simulink library "inp"  (R2021b)
settings: Solver=VariableStepAuto  StartTime=0.0  StopTime=10.0  RelTol=1e-3
undefined symbols (not defined in the file): C_TASK_5MS_S, FALSE, KINP_AcoreReadyToSlp_flg_ovrdflg, KINP_AcoreReadyToSlp_flg_ovrdval, KINP_AllowMovThd_OTA_enum_ovrdflg, KINP_AllowMovThd_OTA_enum_ovrdval, KINP_APSAngleTarget_Deg_ovrdflg, KINP_APSAngleTarget_Deg_ovrdval, KINP_APSDecReq_mps2_ovrdflg, KINP_APSDecReq_mps2_ovrdval, KINP_APSDecReqA_flg_ovrdflg, KINP_APSDecReqA_flg_ovrdval, KINP_APSDFLL_cm_ovrdflg, KINP_APSDFLL_cm_ovrdval, KINP_APSDFLR_cm_ovrdflg, KINP_APSDFLR_cm_ovrdval, KINP_APSDRLL_cm_ovrdflg, KINP_APSDRLL_cm_ovrdval, KINP_APSDRLR_cm_ovrdflg, KINP_APSDRLR_cm_ovrdval, KINP_APSExitCondition_enum_ovrdflg, KINP_APSExitCondition_enum_ovrdval, KINP_APSHWVer_enum_ovrdflg, KINP_APSHWVer_enum_ovrdval, KINP_APSProgressPCT_pct_ovrdflg, KINP_APSProgressPCT_pct_ovrdval, KINP_APSReq_enum_ovrdflg, KINP_APSReq_enum_ovrdval, KINP_APSRQDisplay_enum_ovrdflg, KINP_APSRQDisplay_enum_ovrdval, KINP_APSRqEPASCtrl_flg_ovrdflg, KINP_APSRqEPASCtrl_flg_ovrdval, KINP_APSShiftPosnReq_enum_ovrdval, KINP_APSShiftPosnReq_enum_ovrflg, KINP_APSSpeedCMD_kph_ovrdval, KINP_APSSpeedCMD_kph_ovrflg, KINP_APSStaSystem_enum_ovrdflg, KINP_APSStaSystem_enum_ovrdval, KINP_APSSWVer_enum_ovrdflg, KINP_APSSWVer_enum_ovrdval, KINP_APSVMCReqA_flg_ovrdval, KINP_APSVMCReqA_flg_ovrflg, KINP_APSVRqEPASCtrl_flg_ovrdflg, KINP_APSVRqEPASCtrl_flg_ovrdval, KINP_AuxBattVolmV_mV_ovrdflg, KINP_AuxBattVolmV_mV_ovrdval, KINP_CAASSta_enum_ovrdflg, KINP_CAASSta_enum_ovrdval, KINP_CAASVMCReqA_flg_ovrdval, KINP_CAASVMCReqA_flg_ovrflg, KINP_Chime_enum_ovrdflg, KINP_Chime_enum_ovrdval, KINP_ClearDTCcmd_flg_ovrdflg, KINP_ClearDTCcmd_flg_ovrdval, KINP_EvccAplusPwrUpReq_flg_ovrdflg, KINP_EvccAplusPwrUpReq_flg_ovrdval, KINP_LFID_raw_ovrdval, KINP_LFID_raw_ovrflg, KINP_LRID_raw_ovrdval, KINP_MemOffsetAccX_raw16_ovrdflg ... (+118)
libraries: FVT_lib x595, hcu_lib x1
(part 10 of 27)

== system inp/INP/CAN1/SignalCheck/ESC3 ==
  BHAL_outputs : Inport
  inp_CanValid_bus : Inport  Port=2
  LRPulseCount : FVT_lib/inp/can_signal_template  SystemSampleTime=-1  VariantActivationTime=update diagram  Latency=0  AutoFrameSizeCalculation=off
      link override defval: Value=KINP_LRPulseCount_enum_defval
      link override fftdec: Value=KINP_LRPulseCount_enum_fftdec
      link override fftinc: Value=KINP_LRPulseCount_enum_fftinc
      link override fftlim: Value=KINP_LRPulseCount_enum_fftlim
      link override invalid: Value=KINP_LRPulseCount_enum_invalid
      link override ovrdflg: Value=KINP_LRPulseCount_enum_ovrdflg
      link override ovrdval: Value=KINP_LRPulseCount_enum_ovrdval
      link override setvalid: Value=KINP_LRPulseCount_enum_setvalid
      link override srvcflg: Value=KINP_LRPulseCount_enum_srvcflg
      link override srvcval: Value=KINP_LRPulseCount_enum_srvcval
  LRPulseCountV : FVT_lib/inp/can_signal_template  SystemSampleTime=-1  VariantActivationTime=update diagram  Latency=0  AutoFrameSizeCalculation=off
      link override defval: Value=KINP_LRPulseCountV_flg_defval
      link override fftdec: Value=KINP_LRPulseCountV_flg_fftdec
      link override fftinc: Value=KINP_LRPulseCountV_flg_fftinc
      link override fftlim: Value=KINP_LRPulseCountV_flg_fftlim
      link override invalid: Value=KINP_LRPulseCountV_flg_invalid
      link override ovrdflg: Value=KINP_LRPulseCountV_flg_ovrdflg
      link override ovrdval: Value=KINP_LRPulseCountV_flg_ovrdval
      link override setvalid: Value=KINP_LRPulseCountV_flg_setvalid
      link override srvcflg: Value=KINP_LRPulseCountV_flg_srvcflg
      link override srvcval: Value=KINP_LRPulseCountV_flg_srvcval
  LRRawWhlSpeed : FVT_lib/inp/can_signal_template  SystemSampleTime=-1  VariantActivationTime=update diagram  Latency=0  AutoFrameSizeCalculation=off
      link override defval: Value=KINP_LRRawWhlSpeed_kph_defval
      link override fftdec: Value=KINP_LRRawWhlSpeed_kph_fftdec
      link override fftinc: Value=KINP_LRRawWhlSpeed_kph_fftinc
      link override fftlim: Value=KINP_LRRawWhlSpeed_kph_fftlim
      link override invalid: Value=KINP_LRRawWhlSpeed_kph_invalid
      link override ovrdflg: Value=KINP_LRRawWhlSpeed_kph_ovrdflg
      link override ovrdval: Value=KINP_LRRawWhlSpeed_kph_ovrdval
      link override setvalid: Value=KINP_LRRawWhlSpeed_kph_setvalid
      link override srvcflg: Value=KINP_LRRawWhlSpeed_kph_srvcflg
      link override srvcval: Value=KINP_LRRawWhlSpeed_kph_srvcval
  LRRawWhlSpeedV : FVT_lib/inp/can_signal_template  SystemSampleTime=-1  VariantActivationTime=update diagram  Latency=0  AutoFrameSizeCalculation=off
      link override defval: Value=KINP_LRRawWhlSpeedV_flg_defval
      link override fftdec: Value=KINP_LRRawWhlSpeedV_flg_fftdec
      link override fftinc: Value=KINP_LRRawWhlSpeedV_flg_fftinc
      link override fftlim: Value=KINP_LRRawWhlSpeedV_flg_fftlim
      link override invalid: Value=KINP_LRRawWhlSpeedV_flg_invalid
      link override ovrdflg: Value=KINP_LRRawWhlSpeedV_flg_ovrdflg
      link override ovrdval: Value=KINP_LRRawWhlSpeedV_flg_ovrdval
      link override setvalid: Value=KINP_LRRawWhlSpeedV_flg_setvalid
      link override srvcflg: Value=KINP_LRRawWhlSpeedV_flg_srvcflg
      link override srvcval: Value=KINP_LRRawWhlSpeedV_flg_srvcval
  LRWhlRotDir : FVT_lib/inp/can_signal_template  SystemSampleTime=-1  VariantActivationTime=update diagram  Latency=0  AutoFrameSizeCalculation=off
      link override defval: Value=KINP_LRWhlRotDir_enum_defval
      link override fftdec: Value=KINP_LRWhlRotDir_enum_fftdec
      link override fftinc: Value=KINP_LRWhlRotDir_enum_fftinc
      link override fftlim: Value=KINP_LRWhlRotDir_enum_fftlim
      link override invalid: Value=KINP_LRWhlRotDir_enum_invalid
      link override ovrdflg: Value=KINP_LRWhlRotDir_enum_ovrdflg
      link override ovrdval: Value=KINP_LRWhlRotDir_enum_ovrdval
      link override setvalid: Value=KINP_LRWhlRotDir_enum_setvalid
      link override srvcflg: Value=KINP_LRWhlRotDir_enum_srvcflg
      link override srvcval: Value=KINP_LRWhlRotDir_enum_srvcval
  RRPulseCount : FVT_lib/inp/can_signal_template  SystemSampleTime=-1  VariantActivationTime=update diagram  Latency=0  AutoFrameSizeCalculation=off
      link override defval: Value=KINP_RRPulseCount_enum_defval
      link override fftdec: Value=KINP_RRPulseCount_enum_fftdec
      link override fftinc: Value=KINP_RRPulseCount_enum_fftinc
      link override fftlim: Value=KINP_RRPulseCount_enum_fftlim
      link override invalid: Value=KINP_RRPulseCount_enum_invalid
      link override ovrdflg: Value=KINP_RRPulseCount_enum_ovrdflg
      link override ovrdval: Value=KINP_RRPulseCount_enum_ovrdval
      link override setvalid: Value=KINP_RRPulseCount_enum_setvalid
      link override srvcflg: Value=KINP_RRPulseCount_enum_srvcflg
      link override srvcval: Value=KINP_RRPulseCount_enum_srvcval
  RRPulseCountV : FVT_lib/inp/can_signal_template  SystemSampleTime=-1  VariantActivationTime=update diagram  Latency=0  AutoFrameSizeCalculation=off
      link override defval: Value=KINP_RRPulseCountV_flg_defval
      link override fftdec: Value=KINP_RRPulseCountV_flg_fftdec
      link override fftinc: Value=KINP_RRPulseCountV_flg_fftinc
      link override fftlim: Value=KINP_RRPulseCountV_flg_fftlim
      link override invalid: Value=KINP_RRPulseCountV_flg_invalid
      link override ovrdflg: Value=KINP_RRPulseCountV_flg_ovrdflg
      link override ovrdval: Value=KINP_RRPulseCountV_flg_ovrdval
      link override setvalid: Value=KINP_RRPulseCountV_flg_setvalid
      link override srvcflg: Value=KINP_RRPulseCountV_flg_srvcflg
      link override srvcval: Value=KINP_RRPulseCountV_flg_srvcval
  RRRawWhlSpeed : FVT_lib/inp/can_signal_template  SystemSampleTime=-1  VariantActivationTime=update diagram  Latency=0  AutoFrameSizeCalculation=off
      link override defval: Value=KINP_RRRawWhlSpeed_kph_defval
      link override fftdec: Value=KINP_RRRawWhlSpeed_kph_fftdec
      link override fftinc: Value=KINP_RRRawWhlSpeed_kph_fftinc
      link override fftlim: Value=KINP_RRRawWhlSpeed_kph_fftlim
      link override invalid: Value=KINP_RRRawWhlSpeed_kph_invalid
      link override ovrdflg: Value=KINP_RRRawWhlSpeed_kph_ovrdflg
      link override ovrdval: Value=KINP_RRRawWhlSpeed_kph_ovrdval
      link override setvalid: Value=KINP_RRRawWhlSpeed_kph_setvalid
      link override srvcflg: Value=KINP_RRRawWhlSpeed_kph_srvcflg
      link override srvcval: Value=KINP_RRRawWhlSpeed_kph_srvcval
  RRRawWhlSpeedV : FVT_lib/inp/can_signal_template  SystemSampleTime=-1  VariantActivationTime=update diagram  Latency=0  AutoFrameSizeCalculation=off
      link override defval: Value=KINP_RRRawWhlSpeedV_flg_defval
      link override fftdec: Value=KINP_RRRawWhlSpeedV_flg_fftdec
      link override fftinc: Value=KINP_RRRawWhlSpeedV_flg_fftinc
      link override fftlim: Value=KINP_RRRawWhlSpeedV_flg_fftlim
      link override invalid: Value=KINP_RRRawWhlSpeedV_flg_invalid
      link override ovrdflg: Value=KINP_RRRawWhlSpeedV_flg_ovrdflg
      link override ovrdval: Value=KINP_RRRawWhlSpeedV_flg_ovrdval
      link override setvalid: Value=KINP_RRRawWhlSpeedV_flg_setvalid
      link override srvcflg: Value=KINP_RRRawWhlSpeedV_flg_srvcflg
      link override srvcval: Value=KINP_RRRawWhlSpeedV_flg_srvcval
  RRWhlRotDir : FVT_lib/inp/can_signal_template  SystemSampleTime=-1  VariantActivationTime=update diagram  Latency=0  AutoFrameSizeCalculation=off
      link override defval: Value=KINP_RRWhlRotDir_enum_defval
      link override fftdec: Value=KINP_RRWhlRotDir_enum_fftdec
      link override fftinc: Value=KINP_RRWhlRotDir_enum_fftinc
      link override fftlim: Value=KINP_RRWhlRotDir_enum_fftlim
      link override invalid: Value=KINP_RRWhlRotDir_enum_invalid
      link override ovrdflg: Value=KINP_RRWhlRotDir_enum_ovrdflg
      link override ovrdval: Value=KINP_RRWhlRotDir_enum_ovrdval
      link override setvalid: Value=KINP_RRWhlRotDir_enum_setvalid
      link override srvcflg: Value=KINP_RRWhlRotDir_enum_srvcflg
      link override srvcval: Value=KINP_RRWhlRotDir_enum_srvcval
  Terminator_{1..10} (10 alike) : Terminator
  True_VHAL_LRPulseCountV_flg : Constant  Value=TRUE  OutDataTypeStr=boolean
  True_VHAL_LRPulseCount_enum : Constant  Value=TRUE  OutDataTypeStr=boolean
  True_VHAL_LRRawWhlSpeedV_flg : Constant  Value=TRUE  OutDataTypeStr=boolean
  True_VHAL_LRRawWhlSpeed_kph : Constant  Value=TRUE  OutDataTypeStr=boolean
  True_VHAL_LRWhlRotDir_enum : Constant  Value=TRUE  OutDataTypeStr=boolean
  True_VHAL_RRPulseCountV_flg : Constant  Value=TRUE  OutDataTypeStr=boolean
  True_VHAL_RRPulseCount_enum : Constant  Value=TRUE  OutDataTypeStr=boolean
  True_VHAL_RRRawWhlSpeedV_flg : Constant  Value=TRUE  OutDataTypeStr=boolean
  True_VHAL_RRRawWhlSpeed_kph : Constant  Value=TRUE  OutDataTypeStr=boolean
  True_VHAL_RRWhlRotDir_enum : Constant  Value=TRUE  OutDataTypeStr=boolean
  slr1_{1..10} (10 alike) : BusSelector  OutputSignals=VINP_CANMsgValidESC3_flg
  slr_VHAL_LRPulseCountV_flg : BusSelector  OutputSignals=VHAL_LRPulseCountV_flg
  slr_VHAL_LRPulseCount_enum : BusSelector  OutputSignals=VHAL_LRPulseCount_enum
  slr_VHAL_LRRawWhlSpeedV_flg : BusSelector  OutputSignals=VHAL_LRRawWhlSpeedV_flg
  slr_VHAL_LRRawWhlSpeed_kph : BusSelector  OutputSignals=VHAL_LRRawWhlSpeed_kph
  slr_VHAL_LRWhlRotDir_enum : BusSelector  OutputSignals=VHAL_LRWhlRotDir_enum
  slr_VHAL_RRPulseCountV_flg : BusSelector  OutputSignals=VHAL_RRPulseCountV_flg
  slr_VHAL_RRPulseCount_enum : BusSelector  OutputSignals=VHAL_RRPulseCount_enum
  slr_VHAL_RRRawWhlSpeedV_flg : BusSelector  OutputSignals=VHAL_RRRawWhlSpeedV_flg
  slr_VHAL_RRRawWhlSpeed_kph : BusSelector  OutputSignals=VHAL_RRRawWhlSpeed_kph
  slr_VHAL_RRWhlRotDir_enum : BusSelector  OutputSignals=VHAL_RRWhlRotDir_enum
  VINP_LRPulseCount_enum : Outport
  VINP_LRPulseCountV_flg : Outport  Port=2
  VINP_LRRawWhlSpeed_kph : Outport  Port=3
  VINP_LRRawWhlSpeedV_flg : Outport  Port=4
  VINP_LRWhlRotDir_enum : Outport  Port=5
  VINP_RRPulseCount_enum : Outport  Port=6
  VINP_RRPulseCountV_flg : Outport  Port=7
  VINP_RRRawWhlSpeed_kph : Outport  Port=8
  VINP_RRRawWhlSpeedV_flg : Outport  Port=9
  VINP_RRWhlRotDir_enum : Outport  Port=10
  wires:
  BHAL_outputs/1 -> [BHAL_outputs]
  inp_CanValid_bus/1 -> [inp_CanValid_bus]
  [BHAL_outputs] -> slr_VHAL_LRPulseCount_enum/1
  slr_VHAL_LRPulseCount_enum/1 -> LRPulseCount/1  "<VHAL_LRPulseCount_enum>"
  True_VHAL_LRPulseCount_enum/1 -> LRPulseCount/2
  [inp_CanValid_bus] -> slr1_1/1
  slr1_1/1 -> LRPulseCount/3  "<VINP_CANMsgValidESC3_flg>"
  LRPulseCount/1 -> VINP_LRPulseCount_enum/1  "VINP_LRPulseCount_enum"
  LRPulseCount/2 -> Terminator_1/1
  [BHAL_outputs] -> slr_VHAL_LRPulseCountV_flg/1
  slr_VHAL_LRPulseCountV_flg/1 -> LRPulseCountV/1  "<VHAL_LRPulseCountV_flg>"
  True_VHAL_LRPulseCountV_flg/1 -> LRPulseCountV/2
  [inp_CanValid_bus] -> slr1_2/1
  slr1_2/1 -> LRPulseCountV/3  "<VINP_CANMsgValidESC3_flg>"
  LRPulseCountV/1 -> VINP_LRPulseCountV_flg/1  "VINP_LRPulseCountV_flg"
  LRPulseCountV/2 -> Terminator_2/1
  [BHAL_outputs] -> slr_VHAL_LRRawWhlSpeed_kph/1
  slr_VHAL_LRRawWhlSpeed_kph/1 -> LRRawWhlSpeed/1  "<VHAL_LRRawWhlSpeed_kph>"
  True_VHAL_LRRawWhlSpeed_kph/1 -> LRRawWhlSpeed/2
  [inp_CanValid_bus] -> slr1_3/1
  slr1_3/1 -> LRRawWhlSpeed/3  "<VINP_CANMsgValidESC3_flg>"
  LRRawWhlSpeed/1 -> VINP_LRRawWhlSpeed_kph/1  "VINP_LRRawWhlSpeed_kph"
  LRRawWhlSpeed/2 -> Terminator_3/1
  [BHAL_outputs] -> slr_VHAL_LRRawWhlSpeedV_flg/1
  slr_VHAL_LRRawWhlSpeedV_flg/1 -> LRRawWhlSpeedV/1  "<VHAL_LRRawWhlSpeedV_flg>"
  True_VHAL_LRRawWhlSpeedV_flg/1 -> LRRawWhlSpeedV/2
  [inp_CanValid_bus] -> slr1_4/1
  slr1_4/1 -> LRRawWhlSpeedV/3  "<VINP_CANMsgValidESC3_flg>"
  LRRawWhlSpeedV/1 -> VINP_LRRawWhlSpeedV_flg/1  "VINP_LRRawWhlSpeedV_flg"
  LRRawWhlSpeedV/2 -> Terminator_4/1
  [BHAL_outputs] -> slr_VHAL_LRWhlRotDir_enum/1
  slr_VHAL_LRWhlRotDir_enum/1 -> LRWhlRotDir/1  "<VHAL_LRWhlRotDir_enum>"
  True_VHAL_LRWhlRotDir_enum/1 -> LRWhlRotDir/2
  [inp_CanValid_bus] -> slr1_5/1
  slr1_5/1 -> LRWhlRotDir/3  "<VINP_CANMsgValidESC3_flg>"
  LRWhlRotDir/1 -> VINP_LRWhlRotDir_enum/1  "VINP_LRWhlRotDir_enum"
  LRWhlRotDir/2 -> Terminator_5/1
  [BHAL_outputs] -> slr_VHAL_RRPulseCount_enum/1
  slr_VHAL_RRPulseCount_enum/1 -> RRPulseCount/1  "<VHAL_RRPulseCount_enum>"
  True_VHAL_RRPulseCount_enum/1 -> RRPulseCount/2
  [inp_CanValid_bus] -> slr1_6/1
  slr1_6/1 -> RRPulseCount/3  "<VINP_CANMsgValidESC3_flg>"
  RRPulseCount/1 -> VINP_RRPulseCount_enum/1  "VINP_RRPulseCount_enum"
  RRPulseCount/2 -> Terminator_6/1
  [BHAL_outputs] -> slr_VHAL_RRPulseCountV_flg/1
  slr_VHAL_RRPulseCountV_flg/1 -> RRPulseCountV/1  "<VHAL_RRPulseCountV_flg>"
  True_VHAL_RRPulseCountV_flg/1 -> RRPulseCountV/2
  [inp_CanValid_bus] -> slr1_7/1
  slr1_7/1 -> RRPulseCountV/3  "<VINP_CANMsgValidESC3_flg>"
  RRPulseCountV/1 -> VINP_RRPulseCountV_flg/1  "VINP_RRPulseCountV_flg"
  RRPulseCountV/2 -> Terminator_7/1
  [BHAL_outputs] -> slr_VHAL_RRRawWhlSpeed_kph/1
  slr_VHAL_RRRawWhlSpeed_kph/1 -> RRRawWhlSpeed/1  "<VHAL_RRRawWhlSpeed_kph>"
  True_VHAL_RRRawWhlSpeed_kph/1 -> RRRawWhlSpeed/2
  [inp_CanValid_bus] -> slr1_8/1
  slr1_8/1 -> RRRawWhlSpeed/3  "<VINP_CANMsgValidESC3_flg>"
  RRRawWhlSpeed/1 -> VINP_RRRawWhlSpeed_kph/1  "VINP_RRRawWhlSpeed_kph"
  RRRawWhlSpeed/2 -> Terminator_8/1
  [BHAL_outputs] -> slr_VHAL_RRRawWhlSpeedV_flg/1
  slr_VHAL_RRRawWhlSpeedV_flg/1 -> RRRawWhlSpeedV/1  "<VHAL_RRRawWhlSpeedV_flg>"
  True_VHAL_RRRawWhlSpeedV_flg/1 -> RRRawWhlSpeedV/2
  [inp_CanValid_bus] -> slr1_9/1
  slr1_9/1 -> RRRawWhlSpeedV/3  "<VINP_CANMsgValidESC3_flg>"
  RRRawWhlSpeedV/1 -> VINP_RRRawWhlSpeedV_flg/1  "VINP_RRRawWhlSpeedV_flg"
  RRRawWhlSpeedV/2 -> Terminator_9/1
  [BHAL_outputs] -> slr_VHAL_RRWhlRotDir_enum/1
  slr_VHAL_RRWhlRotDir_enum/1 -> RRWhlRotDir/1  "<VHAL_RRWhlRotDir_enum>"
  True_VHAL_RRWhlRotDir_enum/1 -> RRWhlRotDir/2
  [inp_CanValid_bus] -> slr1_10/1
  slr1_10/1 -> RRWhlRotDir/3  "<VINP_CANMsgValidESC3_flg>"
  RRWhlRotDir/1 -> VINP_RRWhlRotDir_enum/1  "VINP_RRWhlRotDir_enum"
  RRWhlRotDir/2 -> Terminator_10/1

== system inp/INP/CAN1/SignalCheck/ESC4 ==
  BHAL_outputs : Inport
  inp_CanValid_bus : Inport  Port=2
  ABSActive : FVT_lib/inp/can_signal_template  SystemSampleTime=-1  VariantActivationTime=update diagram  Latency=0  AutoFrameSizeCalculation=off
      link override defval: Value=KINP_ABSActive_flg_defval
      link override fftdec: Value=KINP_ABSActive_flg_fftdec
      link override fftinc: Value=KINP_ABSActive_flg_fftinc
      link override fftlim: Value=KINP_ABSActive_flg_fftlim
      link override invalid: Value=KINP_ABSActive_flg_invalid
      link override ovrdflg: Value=KINP_ABSActive_flg_ovrdflg
      link override ovrdval: Value=KINP_ABSActive_flg_ovrdval
      link override setvalid: Value=KINP_ABSActive_flg_setvalid
      link override srvcflg: Value=KINP_ABSActive_flg_srvcflg
      link override srvcval: Value=KINP_ABSActive_flg_srvcval
  ABSFailed : FVT_lib/inp/can_signal_template  SystemSampleTime=-1  VariantActivationTime=update diagram  Latency=0  AutoFrameSizeCalculation=off
      link override defval: Value=KINP_ABSFailed_flg_defval
      link override fftdec: Value=KINP_ABSFailed_flg_fftdec
      link override fftinc: Value=KINP_ABSFailed_flg_fftinc
      link override fftlim: Value=KINP_ABSFailed_flg_fftlim
      link override invalid: Value=KINP_ABSFailed_flg_invalid
      link override ovrdflg: Value=KINP_ABSFailed_flg_ovrdflg
      link override ovrdval: Value=KINP_ABSFailed_flg_ovrdval
      link override setvalid: Value=KINP_ABSFailed_flg_setvalid
      link override srvcflg: Value=KINP_ABSFailed_flg_srvcflg
      link override srvcval: Value=KINP_ABSFailed_flg_srvcval
  AVHActive : FVT_lib/inp/can_signal_template  SystemSampleTime=-1  VariantActivationTime=update diagram  Latency=0  AutoFrameSizeCalculation=off
      link override defval: Value=KINP_AVHActive_flg_defval
      link override fftdec: Value=KINP_AVHActive_flg_fftdec
      link override fftinc: Value=KINP_AVHActive_flg_fftinc
      link override fftlim: Value=KINP_AVHActive_flg_fftlim
      link override invalid: Value=KINP_AVHActive_flg_invalid
      link override ovrdflg: Value=KINP_AVHActive_flg_ovrdflg
      link override ovrdval: Value=KINP_AVHActive_flg_ovrdval
      link override setvalid: Value=KINP_AVHActive_flg_setvalid
      link override srvcflg: Value=KINP_AVHActive_flg_srvcflg
      link override srvcval: Value=KINP_AVHActive_flg_srvcval
  AVHFailed : FVT_lib/inp/can_signal_template  SystemSampleTime=-1  VariantActivationTime=update diagram  Latency=0  AutoFrameSizeCalculation=off
      link override defval: Value=KINP_AVHFailed_flg_defval
      link override fftdec: Value=KINP_AVHFailed_flg_fftdec
      link override fftinc: Value=KINP_AVHFailed_flg_fftinc
      link override fftlim: Value=KINP_AVHFailed_flg_fftlim
      link override invalid: Value=KINP_AVHFailed_flg_invalid
      link override ovrdflg: Value=KINP_AVHFailed_flg_ovrdflg
      link override ovrdval: Value=KINP_AVHFailed_flg_ovrdval
      link override setvalid: Value=KINP_AVHFailed_flg_setvalid
      link override srvcflg: Value=KINP_AVHFailed_flg_srvcflg
      link override srvcval: Value=KINP_AVHFailed_flg_srvcval
  BTCSActive : FVT_lib/inp/can_signal_template  SystemSampleTime=-1  VariantActivationTime=update diagram  Latency=0  AutoFrameSizeCalculation=off
      link override defval: Value=KINP_BTCSActive_flg_defval
      link override fftdec: Value=KINP_BTCSActive_flg_fftdec
      link override fftinc: Value=KINP_BTCSActive_flg_fftinc
      link override fftlim: Value=KINP_BTCSActive_flg_fftlim
      link override invalid: Value=KINP_BTCSActive_flg_invalid
      link override ovrdflg: Value=KINP_BTCSActive_flg_ovrdflg
      link override ovrdval: Value=KINP_BTCSActive_flg_ovrdval
      link override setvalid: Value=KINP_BTCSActive_flg_setvalid
      link override srvcflg: Value=KINP_BTCSActive_flg_srvcflg
      link override srvcval: Value=KINP_BTCSActive_flg_srvcval
  EBDActive : FVT_lib/inp/can_signal_template  SystemSampleTime=-1  VariantActivationTime=update diagram  Latency=0  AutoFrameSizeCalculation=off
      link override defval: Value=KINP_EBDActive_flg_defval
      link override fftdec: Value=KINP_EBDActive_flg_fftdec
      link override fftinc: Value=KINP_EBDActive_flg_fftinc
      link override fftlim: Value=KINP_EBDActive_flg_fftlim
      link override invalid: Value=KINP_EBDActive_flg_invalid
      link override ovrdflg: Value=KINP_EBDActive_flg_ovrdflg
      link override ovrdval: Value=KINP_EBDActive_flg_ovrdval
      link override setvalid: Value=KINP_EBDActive_flg_setvalid
      link override srvcflg: Value=KINP_EBDActive_flg_srvcflg
      link override srvcval: Value=KINP_EBDActive_flg_srvcval
  EBDFailed : FVT_lib/inp/can_signal_template  SystemSampleTime=-1  VariantActivationTime=update diagram  Latency=0  AutoFrameSizeCalculation=off
      link override defval: Value=KINP_EBDFailed_flg_defval
      link override fftdec: Value=KINP_EBDFailed_flg_fftdec
      link override fftinc: Value=KINP_EBDFailed_flg_fftinc
      link override fftlim: Value=KINP_EBDFailed_flg_fftlim
      link override invalid: Value=KINP_EBDFailed_flg_invalid
      link override ovrdflg: Value=KINP_EBDFailed_flg_ovrdflg
      link override ovrdval: Value=KINP_EBDFailed_flg_ovrdval
      link override setvalid: Value=KINP_EBDFailed_flg_setvalid
      link override srvcflg: Value=KINP_EBDFailed_flg_srvcflg
      link override srvcval: Value=KINP_EBDFailed_flg_srvcval
  ESCActive : FVT_lib/inp/can_signal_template  SystemSampleTime=-1  VariantActivationTime=update diagram  Latency=0  AutoFrameSizeCalculation=off
      link override defval: Value=KINP_ESCActive_flg_defval
      link override fftdec: Value=KINP_ESCActive_flg_fftdec
      link override fftinc: Value=KINP_ESCActive_flg_fftinc
      link override fftlim: Value=KINP_ESCActive_flg_fftlim
      link override invalid: Value=KINP_ESCActive_flg_invalid
      link override ovrdflg: Value=KINP_ESCActive_flg_ovrdflg
      link override ovrdval: Value=KINP_ESCActive_flg_ovrdval
      link override setvalid: Value=KINP_ESCActive_flg_setvalid
      link override srvcflg: Value=KINP_ESCActive_flg_srvcflg
      link override srvcval: Value=KINP_ESCActive_flg_srvcval
  ESCFailed : FVT_lib/inp/can_signal_template  SystemSampleTime=-1  VariantActivationTime=update diagram  Latency=0  AutoFrameSizeCalculation=off
      link override defval: Value=KINP_ESCFailed_flg_defval
      link override fftdec: Value=KINP_ESCFailed_flg_fftdec
      link override fftinc: Value=KINP_ESCFailed_flg_fftinc
      link override fftlim: Value=KINP_ESCFailed_flg_fftlim
      link override invalid: Value=KINP_ESCFailed_flg_invalid
      link override ovrdflg: Value=KINP_ESCFailed_flg_ovrdflg
      link override ovrdval: Value=KINP_ESCFailed_flg_ovrdval
      link override setvalid: Value=KINP_ESCFailed_flg_setvalid
      link override srvcflg: Value=KINP_ESCFailed_flg_srvcflg
      link override srvcval: Value=KINP_ESCFailed_flg_srvcval
  ESSActive : FVT_lib/inp/can_signal_template  SystemSampleTime=-1  VariantActivationTime=update diagram  Latency=0  AutoFrameSizeCalculation=off
      link override defval: Value=KINP_ESSActive_flg_defval
      link override fftdec: Value=KINP_ESSActive_flg_fftdec
      link override fftinc: Value=KINP_ESSActive_flg_fftinc
      link override fftlim: Value=KINP_ESSActive_flg_fftlim
      link override invalid: Value=KINP_ESSActive_flg_invalid
      link override ovrdflg: Value=KINP_ESSActive_flg_ovrdflg
      link override ovrdval: Value=KINP_ESSActive_flg_ovrdval
      link override setvalid: Value=KINP_ESSActive_flg_setvalid
      link override srvcflg: Value=KINP_ESSActive_flg_srvcflg
      link override srvcval: Value=KINP_ESSActive_flg_srvcval
  GRADE : FVT_lib/inp/can_signal_template  SystemSampleTime=-1  VariantActivationTime=update diagram  Latency=0  AutoFrameSizeCalculation=off
      link override defval: Value=KINP_GRADE_Deg_defval
      link override fftdec: Value=KINP_GRADE_Deg_fftdec
      link override fftinc: Value=KINP_GRADE_Deg_fftinc
      link override fftlim: Value=KINP_GRADE_Deg_fftlim
      link override invalid: Value=KINP_GRADE_Deg_invalid
      link override ovrdflg: Value=KINP_GRADE_Deg_ovrdflg
      link override ovrdval: Value=KINP_GRADE_Deg_ovrdval
      link override setvalid: Value=KINP_GRADE_Deg_setvalid
      link override srvcflg: Value=KINP_GRADE_Deg_srvcflg
      link override srvcval: Value=KINP_GRADE_Deg_srvcval
  HBBActive : FVT_lib/inp/can_signal_template  SystemSampleTime=-1  VariantActivationTime=update diagram  Latency=0  AutoFrameSizeCalculation=off
      link override defval: Value=KINP_HBBActive_flg_defval
      link override fftdec: Value=KINP_HBBActive_flg_fftdec
      link override fftinc: Value=KINP_HBBActive_flg_fftinc
      link override fftlim: Value=KINP_HBBActive_flg_fftlim
      link override invalid: Value=KINP_HBBActive_flg_invalid
      link override ovrdflg: Value=KINP_HBBActive_flg_ovrdflg
      link override ovrdval: Value=KINP_HBBActive_flg_ovrdval
      link override setvalid: Value=KINP_HBBActive_flg_setvalid
      link override srvcflg: Value=KINP_HBBActive_flg_srvcflg
      link override srvcval: Value=KINP_HBBActive_flg_srvcval
  HBBFailed : FVT_lib/inp/can_signal_template  SystemSampleTime=-1  VariantActivationTime=update diagram  Latency=0  AutoFrameSizeCalculation=off
      link override defval: Value=KINP_HBBFailed_flg_defval
      link override fftdec: Value=KINP_HBBFailed_flg_fftdec
      link override fftinc: Value=KINP_HBBFailed_flg_fftinc
      link override fftlim: Value=KINP_HBBFailed_flg_fftlim
      link override invalid: Value=KINP_HBBFailed_flg_invalid
      link override ovrdflg: Value=KINP_HBBFailed_flg_ovrdflg
      link override ovrdval: Value=KINP_HBBFailed_flg_ovrdval
      link override setvalid: Value=KINP_HBBFailed_flg_setvalid
      link override srvcflg: Value=KINP_HBBFailed_flg_srvcflg
      link override srvcval: Value=KINP_HBBFailed_flg_srvcval
  HDDActive : FVT_lib/inp/can_signal_template  SystemSampleTime=-1  VariantActivationTime=update diagram  Latency=0  AutoFrameSizeCalculation=off
      link override defval: Value=KINP_HDDActive_flg_defval
      link override fftdec: Value=KINP_HDDActive_flg_fftdec
      link override fftinc: Value=KINP_HDDActive_flg_fftinc
      link override fftlim: Value=KINP_HDDActive_flg_fftlim
      link override invalid: Value=KINP_HDDActive_flg_invalid
      link override ovrdflg: Value=KINP_HDDActive_flg_ovrdflg
      link override ovrdval: Value=KINP_HDDActive_flg_ovrdval
      link override setvalid: Value=KINP_HDDActive_flg_setvalid
      link override srvcflg: Value=KINP_HDDActive_flg_srvcflg
      link override srvcval: Value=KINP_HDDActive_flg_srvcval
  HDDFailed : FVT_lib/inp/can_signal_template  SystemSampleTime=-1  VariantActivationTime=update diagram  Latency=0  AutoFrameSizeCalculation=off
      link override defval: Value=KINP_HDDFailed_flg_defval
      link override fftdec: Value=KINP_HDDFailed_flg_fftdec
      link override fftinc: Value=KINP_HDDFailed_flg_fftinc
      link override fftlim: Value=KINP_HDDFailed_flg_fftlim
      link override invalid: Value=KINP_HDDFailed_flg_invalid
      link override ovrdflg: Value=KINP_HDDFailed_flg_ovrdflg
      link override ovrdval: Value=KINP_HDDFailed_flg_ovrdval
      link override setvalid: Value=KINP_HDDFailed_flg_setvalid
      link override srvcflg: Value=KINP_HDDFailed_flg_srvcflg
      link override srvcval: Value=KINP_HDDFailed_flg_srvcval
  HSAActive : FVT_lib/inp/can_signal_template  SystemSampleTime=-1  VariantActivationTime=update diagram  Latency=0  AutoFrameSizeCalculation=off
      link override defval: Value=KINP_HSAActive_flg_defval
      link override fftdec: Value=KINP_HSAActive_flg_fftdec
      link override fftinc: Value=KINP_HSAActive_flg_fftinc
      link override fftlim: Value=KINP_HSAActive_flg_fftlim
      link override invalid: Value=KINP_HSAActive_flg_invalid
      link override ovrdflg: Value=KINP_HSAActive_flg_ovrdflg
      link override ovrdval: Value=KINP_HSAActive_flg_ovrdval
      link override setvalid: Value=KINP_HSAActive_flg_setvalid
      link override srvcflg: Value=KINP_HSAActive_flg_srvcflg
      link override srvcval: Value=KINP_HSAActive_flg_srvcval
  HSAFailed : FVT_lib/inp/can_signal_template  SystemSampleTime=-1  VariantActivationTime=update diagram  Latency=0  AutoFrameSizeCalculation=off
      link override defval: Value=KINP_HSAFailed_flg_defval
      link override fftdec: Value=KINP_HSAFailed_flg_fftdec
      link override fftinc: Value=KINP_HSAFailed_flg_fftinc
      link override fftlim: Value=KINP_HSAFailed_flg_fftlim
      link override invalid: Value=KINP_HSAFailed_flg_invalid
      link override ovrdflg: Value=KINP_HSAFailed_flg_ovrdflg
      link override ovrdval: Value=KINP_HSAFailed_flg_ovrdval
      link override setvalid: Value=KINP_HSAFailed_flg_setvalid
      link override srvcflg: Value=KINP_HSAFailed_flg_srvcflg
      link override srvcval: Value=KINP_HSAFailed_flg_srvcval
  PBAFailed : FVT_lib/inp/can_signal_template  SystemSampleTime=-1  VariantActivationTime=update diagram  Latency=0  AutoFrameSizeCalculation=off
      link override defval: Value=KINP_PBAFailed_flg_defval
      link override fftdec: Value=KINP_PBAFailed_flg_fftdec
      link override fftinc: Value=KINP_PBAFailed_flg_fftinc
      link override fftlim: Value=KINP_PBAFailed_flg_fftlim
      link override invalid: Value=KINP_PBAFailed_flg_invalid
      link override ovrdflg: Value=KINP_PBAFailed_flg_ovrdflg
      link override ovrdval: Value=KINP_PBAFailed_flg_ovrdval
      link override setvalid: Value=KINP_PBAFailed_flg_setvalid
      link override srvcflg: Value=KINP_PBAFailed_flg_srvcflg
      link override srvcval: Value=KINP_PBAFailed_flg_srvcval
  TCSActive : FVT_lib/inp/can_signal_template  SystemSampleTime=-1  VariantActivationTime=update diagram  Latency=0  AutoFrameSizeCalculation=off
      link override defval: Value=KINP_TCSActive_flg_defval
      link override fftdec: Value=KINP_TCSActive_flg_fftdec
      link override fftinc: Value=KINP_TCSActive_flg_fftinc
      link override fftlim: Value=KINP_TCSActive_flg_fftlim
      link override invalid: Value=KINP_TCSActive_flg_invalid
      link override ovrdflg: Value=KINP_TCSActive_flg_ovrdflg
      link override ovrdval: Value=KINP_TCSActive_flg_ovrdval
      link override setvalid: Value=KINP_TCSActive_flg_setvalid
      link override srvcflg: Value=KINP_TCSActive_flg_srvcflg
      link override srvcval: Value=KINP_TCSActive_flg_srvcval
  TCSFailed : FVT_lib/inp/can_signal_template  SystemSampleTime=-1  VariantActivationTime=update diagram  Latency=0  AutoFrameSizeCalculation=off
      link override defval: Value=KINP_TCSFailed_flg_defval
      link override fftdec: Value=KINP_TCSFailed_flg_fftdec
      link override fftinc: Value=KINP_TCSFailed_flg_fftinc
      link override fftlim: Value=KINP_TCSFailed_flg_fftlim
      link override invalid: Value=KINP_TCSFailed_flg_invalid
      link override ovrdflg: Value=KINP_TCSFailed_flg_ovrdflg
      link override ovrdval: Value=KINP_TCSFailed_flg_ovrdval
      link override setvalid: Value=KINP_TCSFailed_flg_setvalid
      link override srvcflg: Value=KINP_TCSFailed_flg_srvcflg
      link override srvcval: Value=KINP_TCSFailed_flg_srvcval
  Terminator_{1..20} (20 alike) : Terminator
  True_VHAL_ABSActive_flg : Constant  Value=TRUE  OutDataTypeStr=boolean
  True_VHAL_ABSFailed_flg : Constant  Value=TRUE  OutDataTypeStr=boolean
  True_VHAL_AVHActive_flg : Constant  Value=TRUE  OutDataTypeStr=boolean
  True_VHAL_AVHFailed_flg : Constant  Value=TRUE  OutDataTypeStr=boolean
  True_VHAL_BTCSActive_flg : Constant  Value=TRUE  OutDataTypeStr=boolean
  True_VHAL_EBDActive_flg : Constant  Value=TRUE  OutDataTypeStr=boolean
  True_VHAL_EBDFailed_flg : Constant  Value=TRUE  OutDataTypeStr=boolean
  True_VHAL_ESCActive_flg : Constant  Value=TRUE  OutDataTypeStr=boolean
  True_VHAL_ESCFailed_flg : Constant  Value=TRUE  OutDataTypeStr=boolean
  True_VHAL_ESSActive_flg : Constant  Value=TRUE  OutDataTypeStr=boolean
  True_VHAL_GRADE_Deg : Constant  Value=TRUE  OutDataTypeStr=boolean
  True_VHAL_HBBActive_flg : Constant  Value=TRUE  OutDataTypeStr=boolean
  True_VHAL_HBBFailed_flg : Constant  Value=TRUE  OutDataTypeStr=boolean
  True_VHAL_HDDActive_flg : Constant  Value=TRUE  OutDataTypeStr=boolean
  True_VHAL_HDDFailed_flg : Constant  Value=TRUE  OutDataTypeStr=boolean
  True_VHAL_HSAActive_flg : Constant  Value=TRUE  OutDataTypeStr=boolean
  True_VHAL_HSAFailed_flg : Constant  Value=TRUE  OutDataTypeStr=boolean
  True_VHAL_PBAFailed_flg : Constant  Value=TRUE  OutDataTypeStr=boolean
  True_VHAL_TCSActive_flg : Constant  Value=TRUE  OutDataTypeStr=boolean
  True_VHAL_TCSFailed_flg : Constant  Value=TRUE  OutDataTypeStr=boolean
  slr1_{1..20} (20 alike) : BusSelector  OutputSignals=VINP_CANMsgValidESC4_flg
  slr_VHAL_ABSActive_flg : BusSelector  OutputSignals=VHAL_ABSActive_flg
  slr_VHAL_ABSFailed_flg : BusSelector  OutputSignals=VHAL_ABSFailed_flg
  slr_VHAL_AVHActive_flg : BusSelector  OutputSignals=VHAL_AVHActive_flg
  slr_VHAL_AVHFailed_flg : BusSelector  OutputSignals=VHAL_AVHFailed_flg
  slr_VHAL_BTCSActive_flg : BusSelector  OutputSignals=VHAL_BTCSActive_flg
  slr_VHAL_EBDActive_flg : BusSelector  OutputSignals=VHAL_EBDActive_flg
  slr_VHAL_EBDFailed_flg : BusSelector  OutputSignals=VHAL_EBDFailed_flg
  slr_VHAL_ESCActive_flg : BusSelector  OutputSignals=VHAL_ESCActive_flg
  slr_VHAL_ESCFailed_flg : BusSelector  OutputSignals=VHAL_ESCFailed_flg
  slr_VHAL_ESSActive_flg : BusSelector  OutputSignals=VHAL_ESSActive_flg
  slr_VHAL_GRADE_Deg : BusSelector  OutputSignals=VHAL_GRADE_Deg
  slr_VHAL_HBBActive_flg : BusSelector  OutputSignals=VHAL_HBBActive_flg
  slr_VHAL_HBBFailed_flg : BusSelector  OutputSignals=VHAL_HBBFailed_flg
  slr_VHAL_HDDActive_flg : BusSelector  OutputSignals=VHAL_HDDActive_flg
  slr_VHAL_HDDFailed_flg : BusSelector  OutputSignals=VHAL_HDDFailed_flg
  slr_VHAL_HSAActive_flg : BusSelector  OutputSignals=VHAL_HSAActive_flg
  slr_VHAL_HSAFailed_flg : BusSelector  OutputSignals=VHAL_HSAFailed_flg
  slr_VHAL_PBAFailed_flg : BusSelector  OutputSignals=VHAL_PBAFailed_flg
  slr_VHAL_TCSActive_flg : BusSelector  OutputSignals=VHAL_TCSActive_flg
  slr_VHAL_TCSFailed_flg : BusSelector  OutputSignals=VHAL_TCSFailed_flg
  VINP_ABSActive_flg : Outport
  VINP_ABSFailed_flg : Outport  Port=2
  VINP_AVHActive_flg : Outport  Port=3
  VINP_AVHFailed_flg : Outport  Port=4
  VINP_BTCSActive_flg : Outport  Port=5
  VINP_EBDActive_flg : Outport  Port=6
  VINP_EBDFailed_flg : Outport  Port=7
  VINP_ESCActive_flg : Outport  Port=8
  VINP_ESCFailed_flg : Outport  Port=9
  VINP_ESSActive_flg : Outport  Port=10
  VINP_GRADE_Deg : Outport  Port=11
  VINP_HBBActive_flg : Outport  Port=12
  VINP_HBBFailed_flg : Outport  Port=13
  VINP_HDDActive_flg : Outport  Port=14
  VINP_HDDFailed_flg : Outport  Port=15
  VINP_HSAActive_flg : Outport  Port=16
  VINP_HSAFailed_flg : Outport  Port=17
  VINP_PBAFailed_flg : Outport  Port=18
  VINP_TCSActive_flg : Outport  Port=19
  VINP_TCSFailed_flg : Outport  Port=20
  wires:
  BHAL_outputs/1 -> [BHAL_outputs]
  inp_CanValid_bus/1 -> [inp_CanValid_bus]
  [BHAL_outputs] -> slr_VHAL_ABSActive_flg/1
  slr_VHAL_ABSActive_flg/1 -> ABSActive/1  "<VHAL_ABSActive_flg>"
  True_VHAL_ABSActive_flg/1 -> ABSActive/2
  [inp_CanValid_bus] -> slr1_1/1
  slr1_1/1 -> ABSActive/3  "<VINP_CANMsgValidESC4_flg>"
  ABSActive/1 -> VINP_ABSActive_flg/1  "VINP_ABSActive_flg"
  ABSActive/2 -> Terminator_1/1
  [BHAL_outputs] -> slr_VHAL_ABSFailed_flg/1
  slr_VHAL_ABSFailed_flg/1 -> ABSFailed/1  "<VHAL_ABSFailed_flg>"
  True_VHAL_ABSFailed_flg/1 -> ABSFailed/2
  [inp_CanValid_bus] -> slr1_2/1
  slr1_2/1 -> ABSFailed/3  "<VINP_CANMsgValidESC4_flg>"
  ABSFailed/1 -> VINP_ABSFailed_flg/1  "VINP_ABSFailed_flg"
  ABSFailed/2 -> Terminator_2/1
  [BHAL_outputs] -> slr_VHAL_AVHActive_flg/1
  slr_VHAL_AVHActive_flg/1 -> AVHActive/1  "<VHAL_AVHActive_flg>"
  True_VHAL_AVHActive_flg/1 -> AVHActive/2
  [inp_CanValid_bus] -> slr1_3/1
  slr1_3/1 -> AVHActive/3  "<VINP_CANMsgValidESC4_flg>"
  AVHActive/1 -> VINP_AVHActive_flg/1  "VINP_AVHActive_flg"
  AVHActive/2 -> Terminator_3/1
  [BHAL_outputs] -> slr_VHAL_AVHFailed_flg/1
  slr_VHAL_AVHFailed_flg/1 -> AVHFailed/1  "<VHAL_AVHFailed_flg>"
  True_VHAL_AVHFailed_flg/1 -> AVHFailed/2
  [inp_CanValid_bus] -> slr1_4/1
  slr1_4/1 -> AVHFailed/3  "<VINP_CANMsgValidESC4_flg>"
  AVHFailed/1 -> VINP_AVHFailed_flg/1  "VINP_AVHFailed_flg"
  AVHFailed/2 -> Terminator_4/1
  [BHAL_outputs] -> slr_VHAL_BTCSActive_flg/1
  slr_VHAL_BTCSActive_flg/1 -> BTCSActive/1  "<VHAL_BTCSActive_flg>"
  True_VHAL_BTCSActive_flg/1 -> BTCSActive/2
  [inp_CanValid_bus] -> slr1_5/1
  slr1_5/1 -> BTCSActive/3  "<VINP_CANMsgValidESC4_flg>"
  BTCSActive/1 -> VINP_BTCSActive_flg/1  "VINP_BTCSActive_flg"
  BTCSActive/2 -> Terminator_5/1
  [BHAL_outputs] -> slr_VHAL_EBDActive_flg/1
  slr_VHAL_EBDActive_flg/1 -> EBDActive/1  "<VHAL_EBDActive_flg>"
  True_VHAL_EBDActive_flg/1 -> EBDActive/2
  [inp_CanValid_bus] -> slr1_6/1
  slr1_6/1 -> EBDActive/3  "<VINP_CANMsgValidESC4_flg>"
  EBDActive/1 -> VINP_EBDActive_flg/1  "VINP_EBDActive_flg"
  EBDActive/2 -> Terminator_6/1
  [BHAL_outputs] -> slr_VHAL_EBDFailed_flg/1
  slr_VHAL_EBDFailed_flg/1 -> EBDFailed/1  "<VHAL_EBDFailed_flg>"
  True_VHAL_EBDFailed_flg/1 -> EBDFailed/2
  [inp_CanValid_bus] -> slr1_7/1
  slr1_7/1 -> EBDFailed/3  "<VINP_CANMsgValidESC4_flg>"
  EBDFailed/1 -> VINP_EBDFailed_flg/1  "VINP_EBDFailed_flg"
  EBDFailed/2 -> Terminator_7/1
  [BHAL_outputs] -> slr_VHAL_ESCActive_flg/1
  slr_VHAL_ESCActive_flg/1 -> ESCActive/1  "<VHAL_ESCActive_flg>"
  True_VHAL_ESCActive_flg/1 -> ESCActive/2
  [inp_CanValid_bus] -> slr1_8/1
  slr1_8/1 -> ESCActive/3  "<VINP_CANMsgValidESC4_flg>"
  ESCActive/1 -> VINP_ESCActive_flg/1  "VINP_ESCActive_flg"
  ESCActive/2 -> Terminator_8/1
  [BHAL_outputs] -> slr_VHAL_ESCFailed_flg/1
  slr_VHAL_ESCFailed_flg/1 -> ESCFailed/1  "<VHAL_ESCFailed_flg>"
  True_VHAL_ESCFailed_flg/1 -> ESCFailed/2
  [inp_CanValid_bus] -> slr1_9/1
  slr1_9/1 -> ESCFailed/3  "<VINP_CANMsgValidESC4_flg>"
  ESCFailed/1 -> VINP_ESCFailed_flg/1  "VINP_ESCFailed_flg"
  ESCFailed/2 -> Terminator_9/1
  [BHAL_outputs] -> slr_VHAL_ESSActive_flg/1
  slr_VHAL_ESSActive_flg/1 -> ESSActive/1  "<VHAL_ESSActive_flg>"
  True_VHAL_ESSActive_flg/1 -> ESSActive/2
  [inp_CanValid_bus] -> slr1_10/1
  slr1_10/1 -> ESSActive/3  "<VINP_CANMsgValidESC4_flg>"
  ESSActive/1 -> VINP_ESSActive_flg/1  "VINP_ESSActive_flg"
  ESSActive/2 -> Terminator_10/1
  [BHAL_outputs] -> slr_VHAL_GRADE_Deg/1
  slr_VHAL_GRADE_Deg/1 -> GRADE/1  "<VHAL_GRADE_Deg>"
  True_VHAL_GRADE_Deg/1 -> GRADE/2
  [inp_CanValid_bus] -> slr1_11/1
  slr1_11/1 -> GRADE/3  "<VINP_CANMsgValidESC4_flg>"
  GRADE/1 -> VINP_GRADE_Deg/1  "VINP_GRADE_Deg"
  GRADE/2 -> Terminator_11/1
  [BHAL_outputs] -> slr_VHAL_HBBActive_flg/1
  slr_VHAL_HBBActive_flg/1 -> HBBActive/1  "<VHAL_HBBActive_flg>"
  True_VHAL_HBBActive_flg/1 -> HBBActive/2
  [inp_CanValid_bus] -> slr1_12/1
  slr1_12/1 -> HBBActive/3  "<VINP_CANMsgValidESC4_flg>"
  HBBActive/1 -> VINP_HBBActive_flg/1  "VINP_HBBActive_flg"
  HBBActive/2 -> Terminator_12/1
  [BHAL_outputs] -> slr_VHAL_HBBFailed_flg/1
  slr_VHAL_HBBFailed_flg/1 -> HBBFailed/1  "<VHAL_HBBFailed_flg>"
  True_VHAL_HBBFailed_flg/1 -> HBBFailed/2
  [inp_CanValid_bus] -> slr1_13/1
  slr1_13/1 -> HBBFailed/3  "<VINP_CANMsgValidESC4_flg>"
  HBBFailed/1 -> VINP_HBBFailed_flg/1  "VINP_HBBFailed_flg"
  HBBFailed/2 -> Terminator_13/1
  [BHAL_outputs] -> slr_VHAL_HDDActive_flg/1
  slr_VHAL_HDDActive_flg/1 -> HDDActive/1  "<VHAL_HDDActive_flg>"
  True_VHAL_HDDActive_flg/1 -> HDDActive/2
  [inp_CanValid_bus] -> slr1_14/1
  slr1_14/1 -> HDDActive/3  "<VINP_CANMsgValidESC4_flg>"
  HDDActive/1 -> VINP_HDDActive_flg/1  "VINP_HDDActive_flg"
  HDDActive/2 -> Terminator_14/1
  [BHAL_outputs] -> slr_VHAL_HDDFailed_flg/1
  slr_VHAL_HDDFailed_flg/1 -> HDDFailed/1  "<VHAL_HDDFailed_flg>"
  True_VHAL_HDDFailed_flg/1 -> HDDFailed/2
  [inp_CanValid_bus] -> slr1_15/1
  slr1_15/1 -> HDDFailed/3  "<VINP_CANMsgValidESC4_flg>"
  HDDFailed/1 -> VINP_HDDFailed_flg/1  "VINP_HDDFailed_flg"
  HDDFailed/2 -> Terminator_15/1
  [BHAL_outputs] -> slr_VHAL_HSAActive_flg/1
  slr_VHAL_HSAActive_flg/1 -> HSAActive/1  "<VHAL_HSAActive_flg>"
  True_VHAL_HSAActive_flg/1 -> HSAActive/2
  [inp_CanValid_bus] -> slr1_16/1
  slr1_16/1 -> HSAActive/3  "<VINP_CANMsgValidESC4_flg>"
  HSAActive/1 -> VINP_HSAActive_flg/1  "VINP_HSAActive_flg"
  HSAActive/2 -> Terminator_16/1
  [BHAL_outputs] -> slr_VHAL_HSAFailed_flg/1
  slr_VHAL_HSAFailed_flg/1 -> HSAFailed/1  "<VHAL_HSAFailed_flg>"
  True_VHAL_HSAFailed_flg/1 -> HSAFailed/2
  [inp_CanValid_bus] -> slr1_17/1
  slr1_17/1 -> HSAFailed/3  "<VINP_CANMsgValidESC4_flg>"
  HSAFailed/1 -> VINP_HSAFailed_flg/1  "VINP_HSAFailed_flg"
  HSAFailed/2 -> Terminator_17/1
  [BHAL_outputs] -> slr_VHAL_PBAFailed_flg/1
  slr_VHAL_PBAFailed_flg/1 -> PBAFailed/1  "<VHAL_PBAFailed_flg>"
  True_VHAL_PBAFailed_flg/1 -> PBAFailed/2
  [inp_CanValid_bus] -> slr1_18/1
  slr1_18/1 -> PBAFailed/3  "<VINP_CANMsgValidESC4_flg>"
  PBAFailed/1 -> VINP_PBAFailed_flg/1  "VINP_PBAFailed_flg"
  PBAFailed/2 -> Terminator_18/1
  [BHAL_outputs] -> slr_VHAL_TCSActive_flg/1
  slr_VHAL_TCSActive_flg/1 -> TCSActive/1  "<VHAL_TCSActive_flg>"
  True_VHAL_TCSActive_flg/1 -> TCSActive/2
  [inp_CanValid_bus] -> slr1_19/1
  slr1_19/1 -> TCSActive/3  "<VINP_CANMsgValidESC4_flg>"
  TCSActive/1 -> VINP_TCSActive_flg/1  "VINP_TCSActive_flg"
  TCSActive/2 -> Terminator_19/1
  [BHAL_outputs] -> slr_VHAL_TCSFailed_flg/1
  slr_VHAL_TCSFailed_flg/1 -> TCSFailed/1  "<VHAL_TCSFailed_flg>"
  True_VHAL_TCSFailed_flg/1 -> TCSFailed/2
  [inp_CanValid_bus] -> slr1_20/1
  slr1_20/1 -> TCSFailed/3  "<VINP_CANMsgValidESC4_flg>"
  TCSFailed/1 -> VINP_TCSFailed_flg/1  "VINP_TCSFailed_flg"
  TCSFailed/2 -> Terminator_20/1
